simulink model "MultiARDroneCtrl"  (R2016b)
settings: Solver=FixedStepAuto  StartTime=0.0  StopTime=inf  FixedStep=sampleTime  RelTol=1e-3  EnableMultiTasking=on
values from neighbouring files (symbols this model uses):
  k_d_xy = 0.1    [start.m]
  k_d_z = 0.1    [start.m]
  k_p_xy = 0.2    [start.m]
  k_p_yaw = 0.5    [start.m]
  k_p_z = 0.8    [start.m]
  limit_cmd_xy = 0.3    [start.m]
  waypoints1 = getWaypoints1()    [start.m]
  waypoints2 = getWaypoints2()    [start.m]
  waypoints3 = getWaypoints3()    [start.m]
undefined symbols (not defined in the file or in its folder): Angular, Linear
libraries: robotlib x15
settings Model: Creator=exbot  LastModifiedBy=zhenglong
settings DataIOCC: LimitDataPoints=on
settings OptimizationCC: MaxStackSize=64
settings DebuggingCC: ParameterTunabilityLossMsg=error  AllowSymbolicDim=off  SFUnexpectedBacktrackingDiag=warning  SFNoUnconditionalDefaultTransitionDiag=warning  SFExecutionAtInitializationDiag=none
settings HardwareCC: ProdBitPerPointer=32  ProdBitPerSizeT=32  ProdBitPerPtrDiffT=32  ProdLargestAtomicFloat=None  ProdIntDivRoundTo=Undefined  ProdEndianess=Unspecified  ProdWordSize=32  ProdHWDeviceType=Generic->Unspecified (assume 32-bit Generic)
settings ModelReferenceCC: PropagateSignalLabelsOutOfModel=off
settings RTWCC: SystemTargetFile=ert.tlc  HardwareBoard=Robot Operating System (ROS)  TLCOptions="-aInlineSetEventsForThisBaseRateFcn=TLC_FALSE -aSuppressMultiTaskScheduler=TLC_FALSE  -aRateBasedStepFcn=0"  TemplateMakefile=ert_default_tmf  Description=Embedded Coder  Toolchain=Catkin  TargetLang=C++
settings CodeAppCC: ForceParamTrailComments=on  IgnoreCustomStorageClasses=off  OperatorAnnotations=on  SimulinkDataObjDesc=on  SFDataObjDesc=on  MATLABFcnDesc=on  InsertBlockDesc=on  MATLABSourceComments=on
settings ERTTargetCC: SupportContinuousTime=on
settings ConfigComp: CovMetricSettings=dw  CovHtmlReporting=on  CovSaveCumulativeToWorkspaceVar=on  CovSaveSingleToWorkspaceVar=on  CovExternalEMLEnable=off

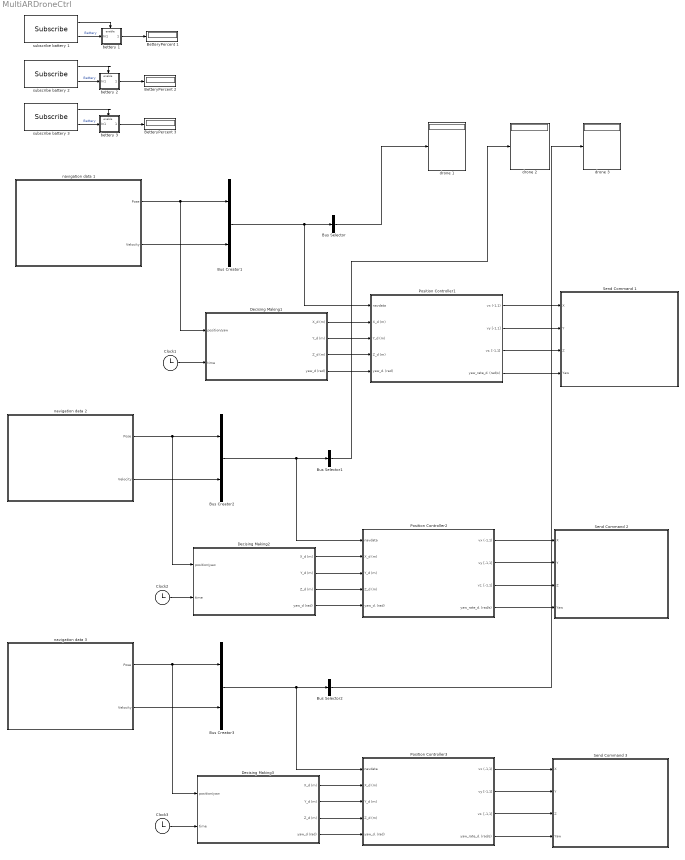
== system MultiARDroneCtrl ==
  BetteryPercent 1 : Display
  BetteryPercent 2 : Display
  BetteryPercent 3 : Display
  Bus Creator1 : BusCreator  Inputs=2
  Bus Creator2 : BusCreator  Inputs=2
  Bus Creator3 : BusCreator  Inputs=2
  Bus Selector : BusSelector  OutputSignals=signal1.x,signal1.y,signal1.z,signal2.vx,signal2.vy,signal2.vz  OutputAsBus=on
  Bus Selector1 : BusSelector  OutputSignals=signal1.x,signal1.y,signal1.z,signal2.vx,signal2.vy,signal2.vz  OutputAsBus=on
  Bus Selector2 : BusSelector  OutputSignals=signal1.x,signal1.y,signal1.z,signal2.vx,signal2.vy,signal2.vz  OutputAsBus=on
  Clock1 : Clock
  Clock2 : Clock
  Clock3 : Clock
  Decising Making1 : Subsystem
  Decising Making2 : Subsystem
  Decising Making3 : Subsystem
  Position Controller1 : Subsystem  AncestorBlock=ARBlocks/Baseline Controller
  Position Controller2 : Subsystem  AncestorBlock=ARBlocks/Baseline Controller
  Position Controller3 : Subsystem  AncestorBlock=ARBlocks/Baseline Controller
  Send Command 1 : Subsystem
  Send Command 2 : Subsystem
  Send Command 3 : Subsystem
  bettery 1 : Subsystem
  bettery 2 : Subsystem
  bettery 3 : Subsystem
  drone 1 : Display
  drone 2 : Display
  drone 3 : Display
  navigation data 1 : Subsystem
  navigation data 2 : Subsystem
  navigation data 3 : Subsystem
  subscribe battery 1 : robotlib/Subscribe  SourceLibraryInfo=This block requires Robotics System Toolbox  topicSource=Specify your own  topic=/ardrone1/ardrone/navdata  messageType=ardrone_autonomy/Navdata  sampleTime=-1  messageQueueLength=1
  subscribe battery 2 : robotlib/Subscribe  SourceLibraryInfo=This block requires Robotics System Toolbox  topicSource=Specify your own  topic=/ardrone2/ardrone/navdata  messageType=ardrone_autonomy/Navdata  sampleTime=-1  messageQueueLength=1
  subscribe battery 3 : robotlib/Subscribe  SourceLibraryInfo=This block requires Robotics System Toolbox  topicSource=Specify your own  topic=/ardrone3/ardrone/navdata  messageType=ardrone_autonomy/Navdata  sampleTime=-1  messageQueueLength=1
  wires:
  Clock1/1 -> Decising Making1/2(time)
  navigation data 1/1(Pose) -> Decising Making1/1(position/yaw), Bus Creator1/1
  navigation data 1/2(Velocity) -> Bus Creator1/2
  Bus Creator1/1 -> Bus Selector/1, Position Controller1/1(navdata)
  Position Controller1/1(vx (-1,1)) -> Send Command 1/1(X)
  Position Controller1/2(vy [-1,1]) -> Send Command 1/2(Y)
  Position Controller1/3(vz. [-1,1]) -> Send Command 1/3(Z)
  Decising Making1/1(X_d (m)) -> Position Controller1/2(X_d (m))
  Decising Making1/2(Y_d (m)) -> Position Controller1/3(Y_d (m))
  Decising Making1/3(Z_d (m)) -> Position Controller1/4(Z_d (m))
  Decising Making1/4(yaw_d (rad)) -> Position Controller1/5(yaw_d. (rad))
  Position Controller1/4(yaw_rate_d. (rad/s)) -> Send Command 1/4(Yaw)
  Clock2/1 -> Decising Making2/2(time)
  navigation data 2/1(Pose) -> Decising Making2/1(position/yaw), Bus Creator2/1
  navigation data 2/2(Velocity) -> Bus Creator2/2
  Position Controller2/1(vx (-1,1)) -> Send Command 2/1(X)
  Position Controller2/2(vy [-1,1]) -> Send Command 2/2(Y)
  Position Controller2/3(vz. [-1,1]) -> Send Command 2/3(Z)
  Decising Making2/1(X_d (m)) -> Position Controller2/2(X_d (m))
  Decising Making2/2(Y_d (m)) -> Position Controller2/3(Y_d (m))
  Decising Making2/3(Z_d (m)) -> Position Controller2/4(Z_d (m))
  Decising Making2/4(yaw_d (rad)) -> Position Controller2/5(yaw_d. (rad))
  Position Controller2/4(yaw_rate_d. (rad/s)) -> Send Command 2/4(Yaw)
  Clock3/1 -> Decising Making3/2(time)
  navigation data 3/1(Pose) -> Decising Making3/1(position/yaw), Bus Creator3/1
  navigation data 3/2(Velocity) -> Bus Creator3/2
  Position Controller3/1(vx (-1,1)) -> Send Command 3/1(X)
  Position Controller3/2(vy [-1,1]) -> Send Command 3/2(Y)
  Position Controller3/3(vz. [-1,1]) -> Send Command 3/3(Z)
  Decising Making3/1(X_d (m)) -> Position Controller3/2(X_d (m))
  Decising Making3/2(Y_d (m)) -> Position Controller3/3(Y_d (m))
  Decising Making3/3(Z_d (m)) -> Position Controller3/4(Z_d (m))
  Decising Making3/4(yaw_d (rad)) -> Position Controller3/5(yaw_d. (rad))
  Position Controller3/4(yaw_rate_d. (rad/s)) -> Send Command 3/4(Yaw)
  Bus Selector/1 -> drone 1/1
  Bus Creator2/1 -> Bus Selector1/1, Position Controller2/1(navdata)
  Bus Selector1/1 -> drone 2/1
  Bus Creator3/1 -> Bus Selector2/1, Position Controller3/1(navdata)
  Bus Selector2/1 -> drone 3/1
  subscribe battery 1/2 -> bettery 1/1(In1)  "Battery"
  subscribe battery 1/1 -> bettery 1/Enable
  bettery 1/1(Out1) -> BetteryPercent 1/1
  subscribe battery 2/2 -> bettery 2/1(In1)  "Battery"
  bettery 2/1(Out1) -> BetteryPercent 2/1
  subscribe battery 2/1 -> bettery 2/Enable
  subscribe battery 3/2 -> bettery 3/1(In1)  "Battery"
  bettery 3/1(Out1) -> BetteryPercent 3/1
  subscribe battery 3/1 -> bettery 3/Enable

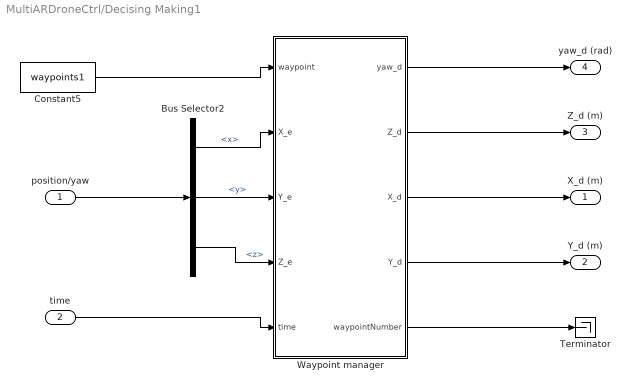
== system MultiARDroneCtrl/Decising Making1 ==
  position/yaw : Inport
  time : Inport  Port=2
  Bus Selector2 : BusSelector  OutputSignals=x,y,z
  Constant5 : Constant  Value=waypoints1  VectorParams1D=off
  Terminator : Terminator
  "Waypoint manager " : MATLAB Function  TreatAsAtomicUnit=on
  X_d (m) : Outport
  Y_d (m) : Outport  Port=2
  Z_d (m) : Outport  Port=3
  yaw_d (rad) : Outport  Port=4
  wires:
  Bus Selector2/1 -> "Waypoint manager "/2(X_e)  "<x>"
  Bus Selector2/2 -> "Waypoint manager "/3(Y_e)  "<y>"
  position/yaw/1 -> Bus Selector2/1
  "Waypoint manager "/2(Z_d) -> Z_d (m)/1
  "Waypoint manager "/3(X_d) -> X_d (m)/1
  "Waypoint manager "/4(Y_d) -> Y_d (m)/1
  time/1 -> "Waypoint manager "/5(time)
  "Waypoint manager "/5(waypointNumber) -> Terminator/1
  "Waypoint manager "/1(yaw_d) -> yaw_d (rad)/1
  Constant5/1 -> "Waypoint manager "/1(waypoint)
  Bus Selector2/3 -> "Waypoint manager "/4(Z_e)  "<z>"

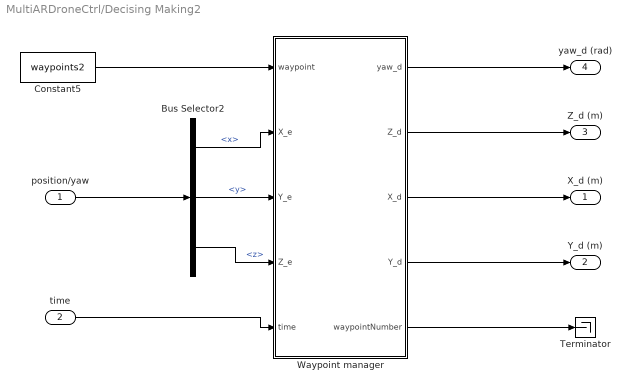
== system MultiARDroneCtrl/Decising Making2 ==
  position/yaw : Inport
  time : Inport  Port=2
  Bus Selector2 : BusSelector  OutputSignals=x,y,z
  Constant5 : Constant  Value=waypoints2  VectorParams1D=off
  Terminator : Terminator
  "Waypoint manager " : MATLAB Function  TreatAsAtomicUnit=on
  X_d (m) : Outport
  Y_d (m) : Outport  Port=2
  Z_d (m) : Outport  Port=3
  yaw_d (rad) : Outport  Port=4
  wires:
  Bus Selector2/1 -> "Waypoint manager "/2(X_e)  "<x>"
  Bus Selector2/2 -> "Waypoint manager "/3(Y_e)  "<y>"
  position/yaw/1 -> Bus Selector2/1
  "Waypoint manager "/2(Z_d) -> Z_d (m)/1
  "Waypoint manager "/3(X_d) -> X_d (m)/1
  "Waypoint manager "/4(Y_d) -> Y_d (m)/1
  time/1 -> "Waypoint manager "/5(time)
  "Waypoint manager "/5(waypointNumber) -> Terminator/1
  "Waypoint manager "/1(yaw_d) -> yaw_d (rad)/1
  Constant5/1 -> "Waypoint manager "/1(waypoint)
  Bus Selector2/3 -> "Waypoint manager "/4(Z_e)  "<z>"

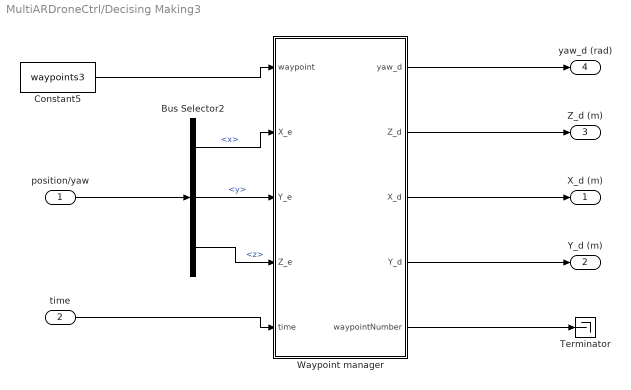
== system MultiARDroneCtrl/Decising Making3 ==
  position/yaw : Inport
  time : Inport  Port=2
  Bus Selector2 : BusSelector  OutputSignals=x,y,z
  Constant5 : Constant  Value=waypoints3  VectorParams1D=off
  Terminator : Terminator
  "Waypoint manager " : MATLAB Function  TreatAsAtomicUnit=on
  X_d (m) : Outport
  Y_d (m) : Outport  Port=2
  Z_d (m) : Outport  Port=3
  yaw_d (rad) : Outport  Port=4
  wires:
  Bus Selector2/1 -> "Waypoint manager "/2(X_e)  "<x>"
  Bus Selector2/2 -> "Waypoint manager "/3(Y_e)  "<y>"
  position/yaw/1 -> Bus Selector2/1
  "Waypoint manager "/2(Z_d) -> Z_d (m)/1
  "Waypoint manager "/3(X_d) -> X_d (m)/1
  "Waypoint manager "/4(Y_d) -> Y_d (m)/1
  time/1 -> "Waypoint manager "/5(time)
  "Waypoint manager "/5(waypointNumber) -> Terminator/1
  "Waypoint manager "/1(yaw_d) -> yaw_d (rad)/1
  Constant5/1 -> "Waypoint manager "/1(waypoint)
  Bus Selector2/3 -> "Waypoint manager "/4(Z_e)  "<z>"

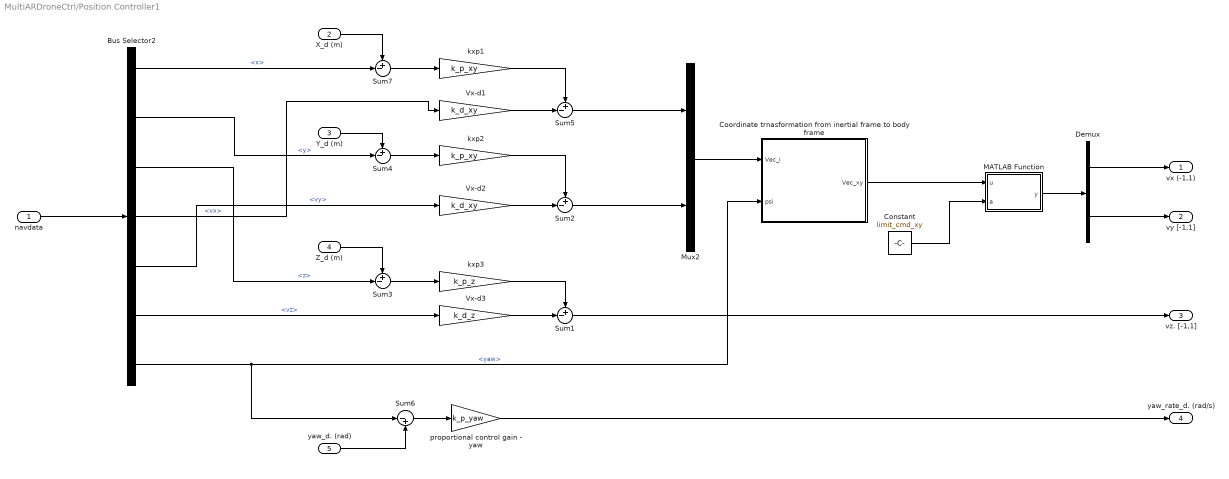
== system MultiARDroneCtrl/Position Controller1 ==
  navdata : Inport
  X_d (m) : Inport  Port=2
  Y_d (m) : Inport  Port=3
  Z_d (m) : Inport  Port=4
  yaw_d. (rad) : Inport  Port=5
  Bus Selector2 : BusSelector  OutputSignals=signal1.x,signal1.y,signal1.z,signal2.vx,signal2.vy,signal2.vz,signal1.yaw
  Constant : Constant  Value=limit_cmd_xy
  "Coordinate trnasformation from inertial frame to body frame " : MATLAB Function  TreatAsAtomicUnit=on
  Demux : Demux  Outputs=2
  MATLAB Function : MATLAB Function  TreatAsAtomicUnit=on
  Mux2 : Mux  Inputs=2
  Sum{1..5,7} (6 alike) : Sum  Inputs=+-|
  Sum6 : Sum  Inputs=|-+
  Vx-d1 : Gain  Gain=k_d_xy
  Vx-d2 : Gain  Gain=k_d_xy
  Vx-d3 : Gain  Gain=k_d_z
  kxp1 : Gain  Gain=k_p_xy
  kxp2 : Gain  Gain=k_p_xy
  kxp3 : Gain  Gain=k_p_z
  proportional control gain - yaw : Gain  Gain=k_p_yaw
  vx (-1,1) : Outport
  vy [-1,1] : Outport  Port=2
  vz. [-1,1] : Outport  Port=3
  yaw_rate_d. (rad/s) : Outport  Port=4
  wires:
  MATLAB Function/1(y) -> Demux/1
  Demux/1 -> vx (-1,1)/1
  Demux/2 -> vy [-1,1]/1
  Constant/1 -> MATLAB Function/2(a)
  Mux2/1 -> "Coordinate trnasformation from inertial frame to body frame "/1(Vec_i)
  Sum7/1 -> kxp1/1
  kxp1/1 -> Sum5/1
  Vx-d1/1 -> Sum5/2
  X_d (m)/1 -> Sum7/1
  Sum4/1 -> kxp2/1
  kxp2/1 -> Sum2/1
  Vx-d2/1 -> Sum2/2
  Y_d (m)/1 -> Sum4/1
  Sum3/1 -> kxp3/1
  kxp3/1 -> Sum1/1
  Vx-d3/1 -> Sum1/2
  Z_d (m)/1 -> Sum3/1
  Bus Selector2/1 -> Sum7/2  "<x>"
  Bus Selector2/2 -> Sum4/2  "<y>"
  Bus Selector2/3 -> Sum3/2  "<z>"
  Bus Selector2/4 -> Vx-d1/1  "<vx>"
  Bus Selector2/5 -> Vx-d2/1  "<vy>"
  Bus Selector2/6 -> Vx-d3/1  "<vz>"
  Bus Selector2/7 -> Sum6/1, "Coordinate trnasformation from inertial frame to body frame "/2(psi)  "<yaw>"
  Sum6/1 -> proportional control gain - yaw/1
  proportional control gain - yaw/1 -> yaw_rate_d. (rad/s)/1
  yaw_d. (rad)/1 -> Sum6/2
  navdata/1 -> Bus Selector2/1
  Sum5/1 -> Mux2/1
  Sum2/1 -> Mux2/2
  Sum1/1 -> vz. [-1,1]/1
  "Coordinate trnasformation from inertial frame to body frame "/1(Vec_xy) -> MATLAB Function/1(u)

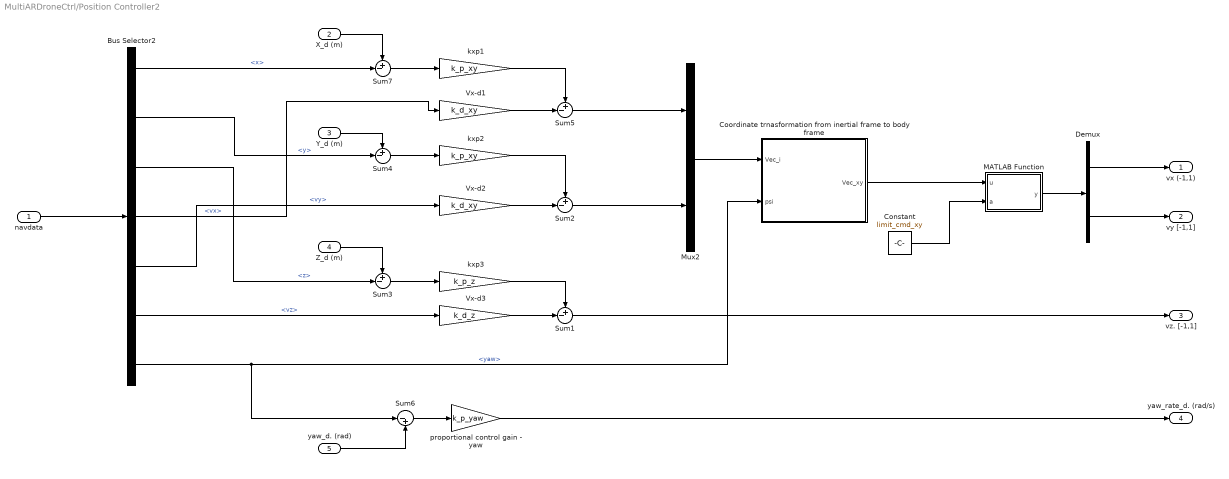
== system MultiARDroneCtrl/Position Controller2 ==
  navdata : Inport
  X_d (m) : Inport  Port=2
  Y_d (m) : Inport  Port=3
  Z_d (m) : Inport  Port=4
  yaw_d. (rad) : Inport  Port=5
  Bus Selector2 : BusSelector  OutputSignals=signal1.x,signal1.y,signal1.z,signal2.vx,signal2.vy,signal2.vz,signal1.yaw
  Constant : Constant  Value=limit_cmd_xy
  "Coordinate trnasformation from inertial frame to body frame " : MATLAB Function  TreatAsAtomicUnit=on
  Demux : Demux  Outputs=2
  MATLAB Function : MATLAB Function  TreatAsAtomicUnit=on
  Mux2 : Mux  Inputs=2
  Sum{1..5,7} (6 alike) : Sum  Inputs=+-|
  Sum6 : Sum  Inputs=|-+
  Vx-d1 : Gain  Gain=k_d_xy
  Vx-d2 : Gain  Gain=k_d_xy
  Vx-d3 : Gain  Gain=k_d_z
  kxp1 : Gain  Gain=k_p_xy
  kxp2 : Gain  Gain=k_p_xy
  kxp3 : Gain  Gain=k_p_z
  proportional control gain - yaw : Gain  Gain=k_p_yaw
  vx (-1,1) : Outport
  vy [-1,1] : Outport  Port=2
  vz. [-1,1] : Outport  Port=3
  yaw_rate_d. (rad/s) : Outport  Port=4
  wires:
  MATLAB Function/1(y) -> Demux/1
  Demux/1 -> vx (-1,1)/1
  Demux/2 -> vy [-1,1]/1
  Constant/1 -> MATLAB Function/2(a)
  Mux2/1 -> "Coordinate trnasformation from inertial frame to body frame "/1(Vec_i)
  Sum7/1 -> kxp1/1
  kxp1/1 -> Sum5/1
  Vx-d1/1 -> Sum5/2
  X_d (m)/1 -> Sum7/1
  Sum4/1 -> kxp2/1
  kxp2/1 -> Sum2/1
  Vx-d2/1 -> Sum2/2
  Y_d (m)/1 -> Sum4/1
  Sum3/1 -> kxp3/1
  kxp3/1 -> Sum1/1
  Vx-d3/1 -> Sum1/2
  Z_d (m)/1 -> Sum3/1
  Bus Selector2/1 -> Sum7/2  "<x>"
  Bus Selector2/2 -> Sum4/2  "<y>"
  Bus Selector2/3 -> Sum3/2  "<z>"
  Bus Selector2/4 -> Vx-d1/1  "<vx>"
  Bus Selector2/5 -> Vx-d2/1  "<vy>"
  Bus Selector2/6 -> Vx-d3/1  "<vz>"
  Bus Selector2/7 -> Sum6/1, "Coordinate trnasformation from inertial frame to body frame "/2(psi)  "<yaw>"
  Sum6/1 -> proportional control gain - yaw/1
  proportional control gain - yaw/1 -> yaw_rate_d. (rad/s)/1
  yaw_d. (rad)/1 -> Sum6/2
  navdata/1 -> Bus Selector2/1
  Sum5/1 -> Mux2/1
  Sum2/1 -> Mux2/2
  Sum1/1 -> vz. [-1,1]/1
  "Coordinate trnasformation from inertial frame to body frame "/1(Vec_xy) -> MATLAB Function/1(u)

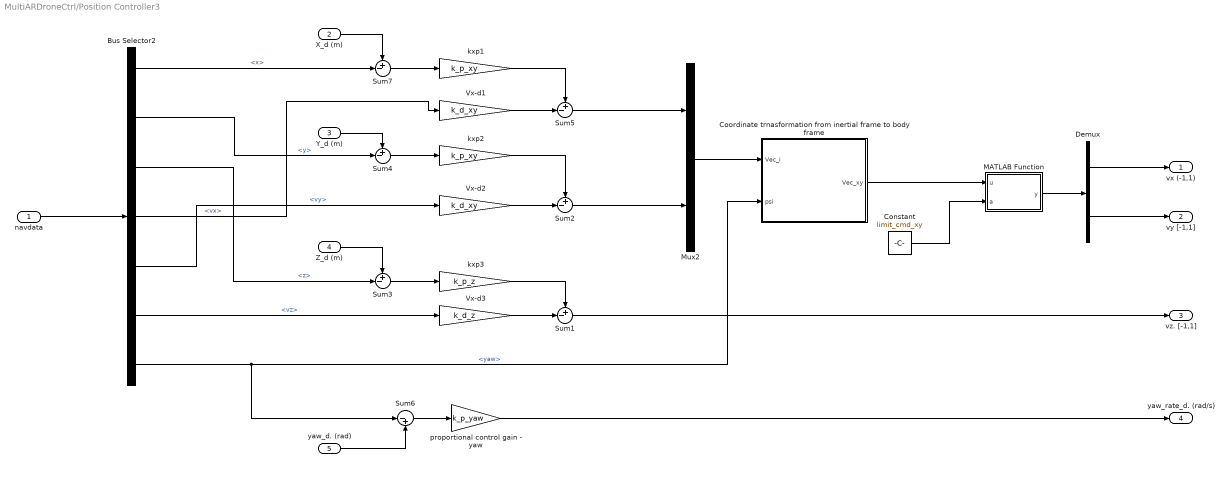
== system MultiARDroneCtrl/Position Controller3 ==
  navdata : Inport
  X_d (m) : Inport  Port=2
  Y_d (m) : Inport  Port=3
  Z_d (m) : Inport  Port=4
  yaw_d. (rad) : Inport  Port=5
  Bus Selector2 : BusSelector  OutputSignals=signal1.x,signal1.y,signal1.z,signal2.vx,signal2.vy,signal2.vz,signal1.yaw
  Constant : Constant  Value=limit_cmd_xy
  "Coordinate trnasformation from inertial frame to body frame " : MATLAB Function  TreatAsAtomicUnit=on
  Demux : Demux  Outputs=2
  MATLAB Function : MATLAB Function  TreatAsAtomicUnit=on
  Mux2 : Mux  Inputs=2
  Sum{1..5,7} (6 alike) : Sum  Inputs=+-|
  Sum6 : Sum  Inputs=|-+
  Vx-d1 : Gain  Gain=k_d_xy
  Vx-d2 : Gain  Gain=k_d_xy
  Vx-d3 : Gain  Gain=k_d_z
  kxp1 : Gain  Gain=k_p_xy
  kxp2 : Gain  Gain=k_p_xy
  kxp3 : Gain  Gain=k_p_z
  proportional control gain - yaw : Gain  Gain=k_p_yaw
  vx (-1,1) : Outport
  vy [-1,1] : Outport  Port=2
  vz. [-1,1] : Outport  Port=3
  yaw_rate_d. (rad/s) : Outport  Port=4
  wires:
  MATLAB Function/1(y) -> Demux/1
  Demux/1 -> vx (-1,1)/1
  Demux/2 -> vy [-1,1]/1
  Constant/1 -> MATLAB Function/2(a)
  Mux2/1 -> "Coordinate trnasformation from inertial frame to body frame "/1(Vec_i)
  Sum7/1 -> kxp1/1
  kxp1/1 -> Sum5/1
  Vx-d1/1 -> Sum5/2
  X_d (m)/1 -> Sum7/1
  Sum4/1 -> kxp2/1
  kxp2/1 -> Sum2/1
  Vx-d2/1 -> Sum2/2
  Y_d (m)/1 -> Sum4/1
  Sum3/1 -> kxp3/1
  kxp3/1 -> Sum1/1
  Vx-d3/1 -> Sum1/2
  Z_d (m)/1 -> Sum3/1
  Bus Selector2/1 -> Sum7/2  "<x>"
  Bus Selector2/2 -> Sum4/2  "<y>"
  Bus Selector2/3 -> Sum3/2  "<z>"
  Bus Selector2/4 -> Vx-d1/1  "<vx>"
  Bus Selector2/5 -> Vx-d2/1  "<vy>"
  Bus Selector2/6 -> Vx-d3/1  "<vz>"
  Bus Selector2/7 -> Sum6/1, "Coordinate trnasformation from inertial frame to body frame "/2(psi)  "<yaw>"
  Sum6/1 -> proportional control gain - yaw/1
  proportional control gain - yaw/1 -> yaw_rate_d. (rad/s)/1
  yaw_d. (rad)/1 -> Sum6/2
  navdata/1 -> Bus Selector2/1
  Sum5/1 -> Mux2/1
  Sum2/1 -> Mux2/2
  Sum1/1 -> vz. [-1,1]/1
  "Coordinate trnasformation from inertial frame to body frame "/1(Vec_xy) -> MATLAB Function/1(u)

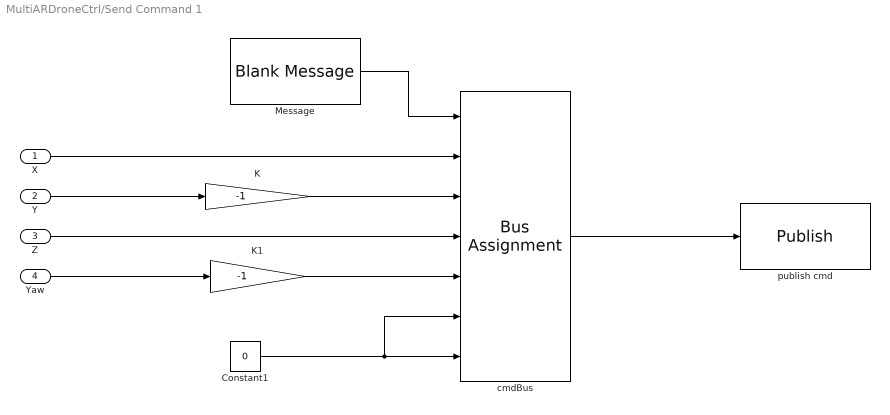
== system MultiARDroneCtrl/Send Command 1 ==
  X : Inport
  Y : Inport  Port=2
  Z : Inport  Port=3
  Yaw : Inport  Port=4
  " Message" : robotlib/Blank Message  SourceLibraryInfo=This block requires Robotics System Toolbox  messageType=geometry_msgs/Twist  SampleTime=inf
  Constant1 : Constant  Value=0
  K : Gain  Gain=-1
  K1 : Gain  Gain=-1
  cmdBus : BusAssignment  AssignedSignals=Linear.X,Linear.Y,Linear.Z,Angular.Z,Angular.X,Angular.Y
  publish cmd : robotlib/Publish  SourceLibraryInfo=This block requires Robotics System Toolbox  topicSource=Select from ROS network  topic=/ardrone1/cmd_vel  messageType=geometry_msgs/Twist  messageQueueLength=1
  wires:
  cmdBus/1 -> publish cmd/1
  Constant1/1 -> cmdBus/6, cmdBus/7
  K/1 -> cmdBus/3
  K1/1 -> cmdBus/5
  " Message"/1 -> cmdBus/1
  X/1 -> cmdBus/2
  Y/1 -> K/1
  Z/1 -> cmdBus/4
  Yaw/1 -> K1/1

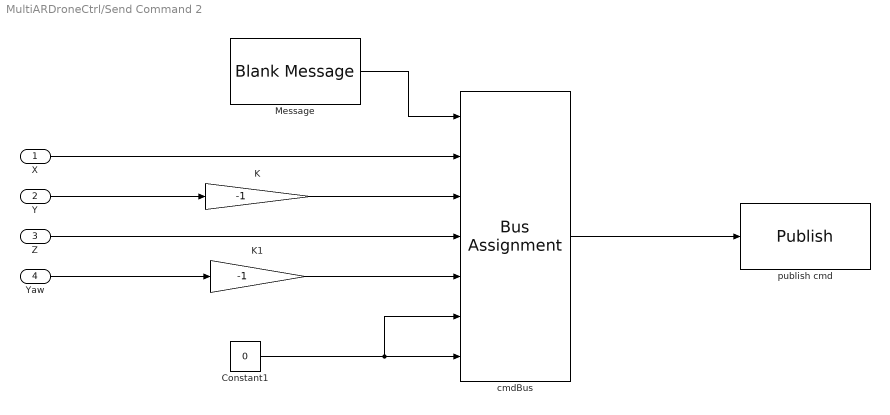
== system MultiARDroneCtrl/Send Command 2 ==
  X : Inport
  Y : Inport  Port=2
  Z : Inport  Port=3
  Yaw : Inport  Port=4
  " Message" : robotlib/Blank Message  SourceLibraryInfo=This block requires Robotics System Toolbox  messageType=geometry_msgs/Twist  SampleTime=inf
  Constant1 : Constant  Value=0
  K : Gain  Gain=-1
  K1 : Gain  Gain=-1
  cmdBus : BusAssignment  AssignedSignals=Linear.X,Linear.Y,Linear.Z,Angular.Z,Angular.X,Angular.Y
  publish cmd : robotlib/Publish  SourceLibraryInfo=This block requires Robotics System Toolbox  topicSource=Select from ROS network  topic=/ardrone2/cmd_vel  messageType=geometry_msgs/Twist  messageQueueLength=1
  wires:
  cmdBus/1 -> publish cmd/1
  Constant1/1 -> cmdBus/6, cmdBus/7
  K/1 -> cmdBus/3
  K1/1 -> cmdBus/5
  " Message"/1 -> cmdBus/1
  X/1 -> cmdBus/2
  Y/1 -> K/1
  Z/1 -> cmdBus/4
  Yaw/1 -> K1/1

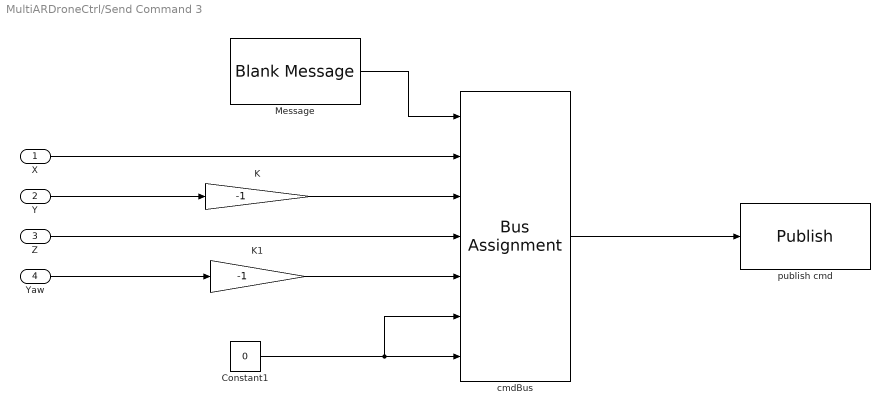
== system MultiARDroneCtrl/Send Command 3 ==
  X : Inport
  Y : Inport  Port=2
  Z : Inport  Port=3
  Yaw : Inport  Port=4
  " Message" : robotlib/Blank Message  SourceLibraryInfo=This block requires Robotics System Toolbox  messageType=geometry_msgs/Twist  SampleTime=inf
  Constant1 : Constant  Value=0
  K : Gain  Gain=-1
  K1 : Gain  Gain=-1
  cmdBus : BusAssignment  AssignedSignals=Linear.X,Linear.Y,Linear.Z,Angular.Z,Angular.X,Angular.Y
  publish cmd : robotlib/Publish  SourceLibraryInfo=This block requires Robotics System Toolbox  topicSource=Select from ROS network  topic=/ardrone3/cmd_vel  messageType=geometry_msgs/Twist  messageQueueLength=1
  wires:
  cmdBus/1 -> publish cmd/1
  Constant1/1 -> cmdBus/6, cmdBus/7
  K/1 -> cmdBus/3
  K1/1 -> cmdBus/5
  " Message"/1 -> cmdBus/1
  X/1 -> cmdBus/2
  Y/1 -> K/1
  Z/1 -> cmdBus/4
  Yaw/1 -> K1/1

== system MultiARDroneCtrl/bettery 1 ==
  In1 : Inport
  Enable : EnablePort
  Bus Selector2 : BusSelector  OutputSignals=BatteryPercent
  Out1 : Outport
  wires:
  In1/1 -> Bus Selector2/1
  Bus Selector2/1 -> Out1/1  "<BatteryPercent>"

== system MultiARDroneCtrl/bettery 2 ==
  In1 : Inport
  Enable : EnablePort
  Bus Selector2 : BusSelector  OutputSignals=BatteryPercent
  Out1 : Outport
  wires:
  In1/1 -> Bus Selector2/1
  Bus Selector2/1 -> Out1/1  "<BatteryPercent>"

== system MultiARDroneCtrl/bettery 3 ==
  In1 : Inport
  Enable : EnablePort
  Bus Selector2 : BusSelector  OutputSignals=BatteryPercent
  Out1 : Outport
  wires:
  In1/1 -> Bus Selector2/1
  Bus Selector2/1 -> Out1/1  "<BatteryPercent>"

== system MultiARDroneCtrl/navigation data 1 ==
  pose : Subsystem
  subscribe pose : robotlib/Subscribe  SourceLibraryInfo=This block requires Robotics System Toolbox  topicSource=Select from ROS network  topic=/Robot_1/pose  messageType=geometry_msgs/PoseStamped  sampleTime=-1  messageQueueLength=1
  subscribe vel : robotlib/Subscribe  SourceLibraryInfo=This block requires Robotics System Toolbox  topicSource=Select from ROS network  topic=/Robot_1/vel  messageType=geometry_msgs/PointStamped  sampleTime=-1  messageQueueLength=1
  vel : Subsystem
  Pose : Outport
  Velocity : Outport  Port=2
  wires:
  subscribe pose/2 -> pose/1(In1)  "position/yaw"
  subscribe pose/1 -> pose/Enable
  subscribe vel/2 -> vel/1(In1)
  subscribe vel/1 -> vel/Enable
  pose/1(Out1) -> Pose/1
  vel/1("Vel ") -> Velocity/1

== system MultiARDroneCtrl/navigation data 2 ==
  pose : Subsystem
  subscribe pose : robotlib/Subscribe  SourceLibraryInfo=This block requires Robotics System Toolbox  topicSource=Select from ROS network  topic=/Robot_2/pose  messageType=geometry_msgs/PoseStamped  sampleTime=-1  messageQueueLength=1
  subscribe vel : robotlib/Subscribe  SourceLibraryInfo=This block requires Robotics System Toolbox  topicSource=Select from ROS network  topic=/Robot_2/vel  messageType=geometry_msgs/PointStamped  sampleTime=-1  messageQueueLength=1
  vel : Subsystem
  Pose : Outport
  Velocity : Outport  Port=2
  wires:
  subscribe pose/2 -> pose/1(In1)  "position/yaw"
  subscribe pose/1 -> pose/Enable
  subscribe vel/2 -> vel/1(In1)
  subscribe vel/1 -> vel/Enable
  pose/1(Out1) -> Pose/1
  vel/1("Vel ") -> Velocity/1

== system MultiARDroneCtrl/navigation data 3 ==
  pose : Subsystem
  subscribe pose : robotlib/Subscribe  SourceLibraryInfo=This block requires Robotics System Toolbox  topicSource=Select from ROS network  topic=/Robot_3/pose  messageType=geometry_msgs/PoseStamped  sampleTime=-1  messageQueueLength=1
  subscribe vel : robotlib/Subscribe  SourceLibraryInfo=This block requires Robotics System Toolbox  topicSource=Select from ROS network  topic=/Robot_3/vel  messageType=geometry_msgs/PointStamped  sampleTime=-1  messageQueueLength=1
  vel : Subsystem
  Pose : Outport
  Velocity : Outport  Port=2
  wires:
  subscribe pose/2 -> pose/1(In1)  "position/yaw"
  subscribe pose/1 -> pose/Enable
  subscribe vel/2 -> vel/1(In1)
  subscribe vel/1 -> vel/Enable
  pose/1(Out1) -> Pose/1
  vel/1("Vel ") -> Velocity/1

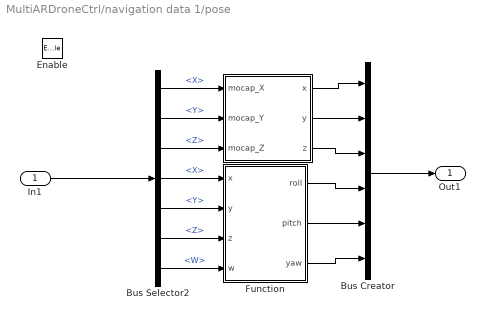
== system MultiARDroneCtrl/navigation data 1/pose ==
  In1 : Inport
  Enable : EnablePort
  " " : MATLAB Function  TreatAsAtomicUnit=on
  " Function" : MATLAB Function  TreatAsAtomicUnit=on
  Bus Creator : BusCreator  Inputs=6
  Bus Selector2 : BusSelector  OutputSignals=Pose.Position.X,Pose.Position.Y,Pose.Position.Z,Pose.Orientation.X,Pose.Orientation.Y,Pose.Orientation.Z,Pose.Orientation.W
  Out1 : Outport
  wires:
  Bus Creator/1 -> Out1/1
  In1/1 -> Bus Selector2/1
  " Function"/1(roll) -> Bus Creator/4
  " Function"/2(pitch) -> Bus Creator/5
  " Function"/3(yaw) -> Bus Creator/6
  Bus Selector2/4 -> " Function"/1(x)  "<X>"
  Bus Selector2/5 -> " Function"/2(y)  "<Y>"
  Bus Selector2/6 -> " Function"/3(z)  "<Z>"
  Bus Selector2/7 -> " Function"/4(w)  "<W>"
  Bus Selector2/1 -> " "/1(mocap_X)  "<X>"
  Bus Selector2/2 -> " "/2(mocap_Y)  "<Y>"
  Bus Selector2/3 -> " "/3(mocap_Z)  "<Z>"
  " "/1(x) -> Bus Creator/1
  " "/2(y) -> Bus Creator/2
  " "/3(z) -> Bus Creator/3

== system MultiARDroneCtrl/navigation data 1/vel ==
  In1 : Inport
  Enable : EnablePort
  " " : MATLAB Function  TreatAsAtomicUnit=on
  Bus Creator : BusCreator  Inputs=3
  Bus Selector2 : BusSelector  OutputSignals=Point.X,Point.Y,Point.Z
  "Vel " : Outport
  wires:
  Bus Creator/1 -> "Vel "/1
  In1/1 -> Bus Selector2/1
  Bus Selector2/1 -> " "/1(mocap_X)  "<X>"
  Bus Selector2/2 -> " "/2(mocap_Y)  "<Y>"
  Bus Selector2/3 -> " "/3(mocap_Z)  "<Z>"
  " "/1(vx) -> Bus Creator/1
  " "/2(vy) -> Bus Creator/2
  " "/3(vz) -> Bus Creator/3

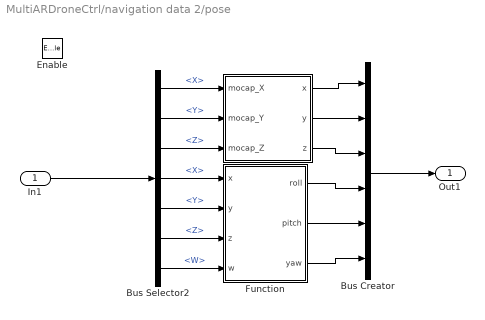
== system MultiARDroneCtrl/navigation data 2/pose ==
  In1 : Inport
  Enable : EnablePort
  " " : MATLAB Function  TreatAsAtomicUnit=on
  " Function" : MATLAB Function  TreatAsAtomicUnit=on
  Bus Creator : BusCreator  Inputs=6
  Bus Selector2 : BusSelector  OutputSignals=Pose.Position.X,Pose.Position.Y,Pose.Position.Z,Pose.Orientation.X,Pose.Orientation.Y,Pose.Orientation.Z,Pose.Orientation.W
  Out1 : Outport
  wires:
  Bus Creator/1 -> Out1/1
  In1/1 -> Bus Selector2/1
  " Function"/1(roll) -> Bus Creator/4
  " Function"/2(pitch) -> Bus Creator/5
  " Function"/3(yaw) -> Bus Creator/6
  Bus Selector2/4 -> " Function"/1(x)  "<X>"
  Bus Selector2/5 -> " Function"/2(y)  "<Y>"
  Bus Selector2/6 -> " Function"/3(z)  "<Z>"
  Bus Selector2/7 -> " Function"/4(w)  "<W>"
  Bus Selector2/1 -> " "/1(mocap_X)  "<X>"
  Bus Selector2/2 -> " "/2(mocap_Y)  "<Y>"
  Bus Selector2/3 -> " "/3(mocap_Z)  "<Z>"
  " "/1(x) -> Bus Creator/1
  " "/2(y) -> Bus Creator/2
  " "/3(z) -> Bus Creator/3

== system MultiARDroneCtrl/navigation data 2/vel ==
  In1 : Inport
  Enable : EnablePort
  " " : MATLAB Function  TreatAsAtomicUnit=on
  Bus Creator : BusCreator  Inputs=3
  Bus Selector2 : BusSelector  OutputSignals=Point.X,Point.Y,Point.Z
  "Vel " : Outport
  wires:
  Bus Creator/1 -> "Vel "/1
  In1/1 -> Bus Selector2/1
  Bus Selector2/1 -> " "/1(mocap_X)  "<X>"
  Bus Selector2/2 -> " "/2(mocap_Y)  "<Y>"
  Bus Selector2/3 -> " "/3(mocap_Z)  "<Z>"
  " "/1(vx) -> Bus Creator/1
  " "/2(vy) -> Bus Creator/2
  " "/3(vz) -> Bus Creator/3

== system MultiARDroneCtrl/navigation data 3/pose ==
  In1 : Inport
  Enable : EnablePort
  " " : MATLAB Function  TreatAsAtomicUnit=on
  " Function" : MATLAB Function  TreatAsAtomicUnit=on
  Bus Creator : BusCreator  Inputs=6
  Bus Selector2 : BusSelector  OutputSignals=Pose.Position.X,Pose.Position.Y,Pose.Position.Z,Pose.Orientation.X,Pose.Orientation.Y,Pose.Orientation.Z,Pose.Orientation.W
  Out1 : Outport
  wires:
  Bus Creator/1 -> Out1/1
  In1/1 -> Bus Selector2/1
  " Function"/1(roll) -> Bus Creator/4
  " Function"/2(pitch) -> Bus Creator/5
  " Function"/3(yaw) -> Bus Creator/6
  Bus Selector2/4 -> " Function"/1(x)  "<X>"
  Bus Selector2/5 -> " Function"/2(y)  "<Y>"
  Bus Selector2/6 -> " Function"/3(z)  "<Z>"
  Bus Selector2/7 -> " Function"/4(w)  "<W>"
  Bus Selector2/1 -> " "/1(mocap_X)  "<X>"
  Bus Selector2/2 -> " "/2(mocap_Y)  "<Y>"
  Bus Selector2/3 -> " "/3(mocap_Z)  "<Z>"
  " "/1(x) -> Bus Creator/1
  " "/2(y) -> Bus Creator/2
  " "/3(z) -> Bus Creator/3

== system MultiARDroneCtrl/navigation data 3/vel ==
  In1 : Inport
  Enable : EnablePort
  " " : MATLAB Function  TreatAsAtomicUnit=on
  Bus Creator : BusCreator  Inputs=3
  Bus Selector2 : BusSelector  OutputSignals=Point.X,Point.Y,Point.Z
  "Vel " : Outport
  wires:
  Bus Creator/1 -> "Vel "/1
  In1/1 -> Bus Selector2/1
  Bus Selector2/1 -> " "/1(mocap_X)  "<X>"
  Bus Selector2/2 -> " "/2(mocap_Y)  "<Y>"
  Bus Selector2/3 -> " "/3(mocap_Z)  "<Z>"
  " "/1(vx) -> Bus Creator/1
  " "/2(vy) -> Bus Creator/2
  " "/3(vz) -> Bus Creator/3

== matlab function MultiARDroneCtrl/Decising Making2/Waypoint manager  ==
  data: yaw_d output; Z_d output; waypoint input; X_e input; Y_e input; Z_e input; X_d output; Y_d output; time input; waypointNumber output
function [yaw_d, Z_d,  X_d, Y_d, waypointNumber]       = fcn(waypoint, X_e,Y_e,Z_e,time )
nPoints = size(waypoint, 2) ;
persistent wpointer;
persistent t0 ;

if isempty(wpointer)
    wpointer = 1;
end
if(wpointer == nPoints)
    disp('The flight task is finished!');
end
if isempty(t0)
    t0 = 0;
end

if ( norm([X_e,Y_e,Z_e]' - waypoint(1:3, wpointer) )< 0.3) 
    yaw_d = waypoint(4, wpointer) ;
    % 当飞机进入目标航路点时，
    % 开始把当前航路点的期望偏航角赋值给控制器，
    % 控制机头指向下一个航路点
    if(wpointer ~= nPoints)        
        if (t0 ==0)
            t0 = time;
        else
            if ((time - t0 > waypoint(5, wpointer)))  % 严格来说飞机在当前航路点的悬停时间
                                                                                   % 应该要足以把偏航角控制到位
                                                                                   % 或者在判断语句中加入偏航角控制到位的判断
                 if(wpointer < nPoints)
                    wpointer = wpointer+ 1;
                    t0 = 0;
                 else
                    disp('The flight task is finished!'); 
                    disp('The flight task is finished!');
                    disp('The flight task is finished!');
                    disp('The flight task is finished!');
                    disp('The flight task is finished!');
                 end
            
            end
        end         
    end    
else  % 如果飞机离开当前航路点，飞向下一个航路点，waypoint
          % 应该继续把当前航路点的期望偏航角赋值给控制器，waypoint
          % 因为飞机需要在飞行过程中继续指向下一个航路点
    if(wpointer>1)
        yaw_d = waypoint(4, wpointer-1) ;
    else
        yaw_d = 0;
    end
end
%% Outputs
Z_d =  waypoint(3, wpointer);
%Z_d = 1.2;
X_d = waypoint(1, wpointer) ;
Y_d = waypoint(2, wpointer) ;
waypointNumber = wpointer ;

== matlab function MultiARDroneCtrl/Decising Making1/Waypoint manager  ==
  data: yaw_d output; Z_d output; waypoint input; X_e input; Y_e input; Z_e input; X_d output; Y_d output; time input; waypointNumber output
function [yaw_d, Z_d,  X_d, Y_d, waypointNumber]       = fcn(waypoint, X_e,Y_e,Z_e,time )
nPoints = size(waypoint, 2) ;
persistent wpointer;
persistent t0 ;

if isempty(wpointer)
    wpointer = 1;
end

if(wpointer == nPoints)
    disp('The flight task is finished!');
end

if isempty(t0)
    t0 = 0;
end

if ( norm([X_e,Y_e,Z_e]' - waypoint(1:3, wpointer) )< 0.3) 
    yaw_d = waypoint(4, wpointer) ;
    % 当飞机进入目标航路点时，
    % 开始把当前航路点的期望偏航角赋值给控制器，
    % 控制机头指向下一个航路点
    if(wpointer ~= nPoints)        
        if (t0 ==0)
            t0 = time;
        else
            if ((time - t0 > waypoint(5, wpointer)))  % 严格来说飞机在当前航路点的悬停时间
                                                                                   % 应该要足以把偏航角控制到位
                                                                                   % 或者在判断语句中加入偏航角控制到位的判断
                 if(wpointer < nPoints)
                    wpointer = wpointer+ 1;
                    t0 = 0;
                 else
                    disp('The flight task is finished!'); 
                    disp('The flight task is finished!');
                    disp('The flight task is finished!');
                    disp('The flight task is finished!');
                    disp('The flight task is finished!');
                 end
            
            end
        end         
    end    
else  % 如果飞机离开当前航路点，飞向下一个航路点，waypoint
          % 应该继续把当前航路点的期望偏航角赋值给控制器，waypoint
          % 因为飞机需要在飞行过程中继续指向下一个航路点
    if(wpointer>1)
        yaw_d = waypoint(4, wpointer-1) ;
    else
        yaw_d = 0;
    end
     
end
%% Outputs
Z_d =  waypoint(3, wpointer);
%Z_d = 1.2;
X_d = waypoint(1, wpointer) ;
Y_d = waypoint(2, wpointer) ;
waypointNumber = wpointer ;

== matlab function MultiARDroneCtrl/navigation data 1/pose/  ==
  data: x output; mocap_X input; y output; mocap_Y input; mocap_Z input; z output
function [x, y, z] = xyz_tf(mocap_X, mocap_Y, mocap_Z)
x = - mocap_Y;
y = - mocap_X;
z = mocap_Z;

== matlab function MultiARDroneCtrl/navigation data 1/pose/ Function ==
  data: x input; roll output; y input; z input; w input; pitch output; yaw output
function [roll, pitch, yaw] = quat2rpy(x, y, z, w)
    t0 = -2.0 * (y * y + z * z) + 1.0;
    t1 = +2.0 * (x * y + w * z);
    t2 = -2.0 * (x * z - w * y);
    t3 = +2.0 * (y * z + w * x);
    t4 = -2.0 * (x * x + y * y) + 1.0;

    roll = -asin(t2);
    pitch = -atan2(t3, t4);
    yaw= -atan2(t1, t0);

== matlab function MultiARDroneCtrl/Position Controller1/MATLAB Function ==
  data: u input; y output; a input
function y = fcn(u,a)
y = satgd(u,a);

== matlab function MultiARDroneCtrl/Decising Making3/Waypoint manager  ==
  data: yaw_d output; Z_d output; waypoint input; X_e input; Y_e input; Z_e input; X_d output; Y_d output; time input; waypointNumber output
function [yaw_d, Z_d,  X_d, Y_d, waypointNumber]       = fcn(waypoint, X_e,Y_e,Z_e,time )
nPoints = size(waypoint, 2) ;
persistent wpointer;
persistent t0 ;

if isempty(wpointer)
    wpointer = 1;
end
if(wpointer == nPoints)
    disp('The flight task is finished!');
end
if isempty(t0)
    t0 = 0;
end

if ( norm([X_e,Y_e,Z_e]' - waypoint(1:3, wpointer) )< 0.3) 
    yaw_d = waypoint(4, wpointer) ;
    % 当飞机进入目标航路点时，
    % 开始把当前航路点的期望偏航角赋值给控制器，
    % 控制机头指向下一个航路点
    if(wpointer ~= nPoints)        
        if (t0 ==0)
            t0 = time;
        else
            if ((time - t0 > waypoint(5, wpointer)))  % 严格来说飞机在当前航路点的悬停时间
                                                                                   % 应该要足以把偏航角控制到位
                                                                                   % 或者在判断语句中加入偏航角控制到位的判断
                 if(wpointer < nPoints)
                    wpointer = wpointer+ 1;
                    t0 = 0;
                 else
                    disp('The flight task is finished!'); 
                    disp('The flight task is finished!');
                    disp('The flight task is finished!');
                    disp('The flight task is finished!');
                    disp('The flight task is finished!');
                 end
            
            end
        end         
    end    
else  % 如果飞机离开当前航路点，飞向下一个航路点，waypoint
          % 应该继续把当前航路点的期望偏航角赋值给控制器，waypoint
          % 因为飞机需要在飞行过程中继续指向下一个航路点
    if(wpointer>1)
        yaw_d = waypoint(4, wpointer-1) ;
    else
        yaw_d = 0;
    end
end
%% Outputs
Z_d =  waypoint(3, wpointer);
%Z_d = 1.2;
X_d = waypoint(1, wpointer) ;
Y_d = waypoint(2, wpointer) ;
waypointNumber = wpointer ;

== matlab function MultiARDroneCtrl/navigation data 1/vel/  ==
  data: vx output; mocap_X input; vy output; mocap_Y input; mocap_Z input; vz output
function [vx, vy, vz] = xyz_tf(mocap_X, mocap_Y, mocap_Z)
vx = - mocap_Y;
vy = - mocap_X;
vz = mocap_Z;

== matlab function MultiARDroneCtrl/Position Controller2/Coordinate trnasformation from inertial frame to body frame  ==
  data: Vec_i input; Vec_xy output; psi input
function Vec_xy  = fcn(Vec_i , psi)
%#codegen
T = [cos(psi) sin(psi) ; -sin(psi) cos(psi)] ; 
Vec_xy = T*Vec_i(1:2,1);

== matlab function MultiARDroneCtrl/Position Controller2/MATLAB Function ==
  data: u input; y output; a input
function y = fcn(u,a)
y = satgd(u,a);

== matlab function MultiARDroneCtrl/navigation data 2/pose/  ==
  data: x output; mocap_X input; y output; mocap_Y input; mocap_Z input; z output
function [x, y, z] = xyz_tf(mocap_X, mocap_Y, mocap_Z)
x = - mocap_Y;
y = - mocap_X;
z = mocap_Z;

== matlab function MultiARDroneCtrl/navigation data 2/pose/ Function ==
  data: x input; roll output; y input; z input; w input; pitch output; yaw output
function [roll, pitch, yaw] = quat2rpy(x, y, z, w)
    t0 = -2.0 * (y * y + z * z) + 1.0;
    t1 = +2.0 * (x * y + w * z);
    t2 = -2.0 * (x * z - w * y);
    t3 = +2.0 * (y * z + w * x);
    t4 = -2.0 * (x * x + y * y) + 1.0;

    roll = -asin(t2);
    pitch = -atan2(t3, t4);
    yaw= -atan2(t1, t0);

== matlab function MultiARDroneCtrl/navigation data 2/vel/  ==
  data: vx output; mocap_X input; vy output; mocap_Y input; mocap_Z input; vz output
function [vx, vy, vz] = xyz_tf(mocap_X, mocap_Y, mocap_Z)
vx = - mocap_Y;
vy = - mocap_X;
vz = mocap_Z;

== matlab function MultiARDroneCtrl/Position Controller1/Coordinate trnasformation from inertial frame to body frame  ==
  data: Vec_i input; Vec_xy output; psi input
function Vec_xy  = fcn(Vec_i , psi)
%#codegen
T = [cos(psi) sin(psi) ; -sin(psi) cos(psi)] ; 
Vec_xy = T*Vec_i(1:2,1);

== matlab function MultiARDroneCtrl/Position Controller3/Coordinate trnasformation from inertial frame to body frame  ==
  data: Vec_i input; Vec_xy output; psi input
function Vec_xy  = fcn(Vec_i , psi)
%#codegen
T = [cos(psi) sin(psi) ; -sin(psi) cos(psi)] ; 
Vec_xy = T*Vec_i(1:2,1);

== matlab function MultiARDroneCtrl/Position Controller3/MATLAB Function ==
  data: u input; y output; a input
function y = fcn(u,a)
y = satgd(u,a);

== matlab function MultiARDroneCtrl/navigation data 3/pose/  ==
  data: x output; mocap_X input; y output; mocap_Y input; mocap_Z input; z output
function [x, y, z] = xyz_tf(mocap_X, mocap_Y, mocap_Z)
x = - mocap_Y;
y = - mocap_X;
z = mocap_Z;

== matlab function MultiARDroneCtrl/navigation data 3/pose/ Function ==
  data: x input; roll output; y input; z input; w input; pitch output; yaw output
function [roll, pitch, yaw] = quat2rpy(x, y, z, w)
    t0 = -2.0 * (y * y + z * z) + 1.0;
    t1 = +2.0 * (x * y + w * z);
    t2 = -2.0 * (x * z - w * y);
    t3 = +2.0 * (y * z + w * x);
    t4 = -2.0 * (x * x + y * y) + 1.0;

    roll = -asin(t2);
    pitch = -atan2(t3, t4);
    yaw= -atan2(t1, t0);

== matlab function MultiARDroneCtrl/navigation data 3/vel/  ==
  data: vx output; mocap_X input; vy output; mocap_Y input; mocap_Z input; vz output
function [vx, vy, vz] = xyz_tf(mocap_X, mocap_Y, mocap_Z)
vx = - mocap_Y;
vy = - mocap_X;
vz = mocap_Z;
